simulink model "target_generation_lib_test"  (R2018b)
settings: Solver=VariableStepAuto  StartTime=0.0  StopTime=10.0  RelTol=1e-3
undefined symbols (not defined in the file): fswParams
libraries: sharedutil x2, sharedtransform x2, target_gen_lib x1
settings Model: Creator=taylorreynolds  LastModifiedBy=taylorreynolds

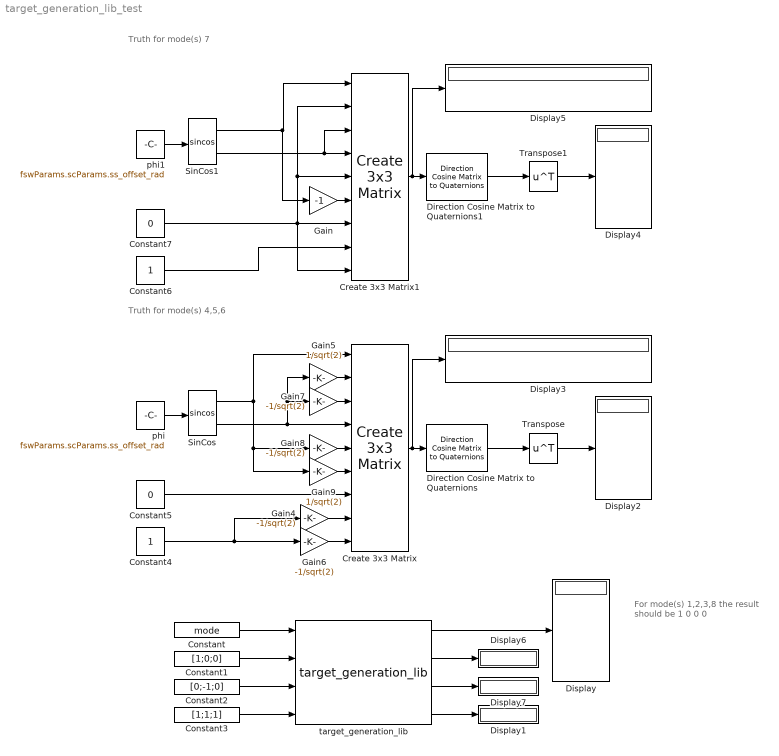
== system target_generation_lib_test ==
  note: For mode(s) 1,2,3,8
      | the result should be
      | 1
      | 0
      | 0
      | 0
  note: Truth for mode(s) 7
  note: Truth for mode(s) 4,5,6
  Constant : Constant  Value=mode  mask{mode=6}
      mask prompts: mode "Choose gnc_mode"
      mask TypeOptions mode: 1 | 2 | 3 | 4 | 5 | 6 | 7 | 8
  Constant1 : Constant  Value=[1;0;0]
  Constant2 : Constant  Value=[0;-1;0]
  Constant3 : Constant  Value=[1;1;1]
  Constant4 : Constant
  Constant5 : Constant  Value=0
  Constant6 : Constant
  Constant7 : Constant  Value=0
  Create 3x3 Matrix : sharedutil/Create 3x3 Matrix  aMode=aMode
  Create 3x3 Matrix1 : sharedutil/Create 3x3 Matrix  aMode=aMode
  Direction Cosine Matrix to Quaternions : sharedtransform/Direction Cosine Matrix  to Quaternions  aMode=0  action=None  tolerance=eps(2)
      settings: SourceProductName=Aerospace Blockset  SourceProductBaseCode=AE
  Direction Cosine Matrix to Quaternions1 : sharedtransform/Direction Cosine Matrix  to Quaternions  aMode=0  action=None  tolerance=eps(2)
      settings: SourceProductName=Aerospace Blockset  SourceProductBaseCode=AE
  Display{,1..7} (8 alike) : Display
  Gain : Gain  Gain=-1
  Gain{4,6..8} (4 alike) : Gain  Gain=-1/sqrt(2)
  Gain5 : Gain  Gain=1/sqrt(2)
  Gain9 : Gain  Gain=1/sqrt(2)
  SinCos : Trigonometry  Operator=sincos
  SinCos1 : Trigonometry  Operator=sincos
  Transpose : Math  Operator=transpose  SaturateOnIntegerOverflow=on
  Transpose1 : Math  Operator=transpose  SaturateOnIntegerOverflow=on
  phi : Constant  Value=fswParams.scParams.ss_offset_rad
  phi1 : Constant  Value=fswParams.scParams.ss_offset_rad
  target_generation_lib : target_gen_lib/target_generation_lib  SystemSampleTime=-1
  wires:
  target_generation_lib/1 -> Display/1
  target_generation_lib/4 -> Display1/1
  Constant/1 -> target_generation_lib/1
  Constant1/1 -> target_generation_lib/2
  Constant2/1 -> target_generation_lib/3
  Constant3/1 -> target_generation_lib/4
  Create 3x3 Matrix/1 -> Display3/1, Direction Cosine Matrix to Quaternions/1
  SinCos/1 -> Gain9/1, Gain8/1, Create 3x3 Matrix/1
  Constant4/1 -> Gain4/1, Gain6/1
  Transpose/1 -> Display2/1
  Direction Cosine Matrix to Quaternions/1 -> Transpose/1
  SinCos/2 -> Gain7/1, Gain5/1, Create 3x3 Matrix/4
  Gain8/1 -> Create 3x3 Matrix/5
  Gain7/1 -> Create 3x3 Matrix/3
  Gain4/1 -> Create 3x3 Matrix/8
  Constant5/1 -> Create 3x3 Matrix/7
  Gain5/1 -> Create 3x3 Matrix/2
  Gain6/1 -> Create 3x3 Matrix/9
  phi/1 -> SinCos/1
  Gain9/1 -> Create 3x3 Matrix/6
  Create 3x3 Matrix1/1 -> Display5/1, Direction Cosine Matrix to Quaternions1/1
  SinCos1/1 -> Gain/1, Create 3x3 Matrix1/1
  Constant6/1 -> Create 3x3 Matrix1/8
  Transpose1/1 -> Display4/1
  Direction Cosine Matrix to Quaternions1/1 -> Transpose1/1
  phi1/1 -> SinCos1/1
  Constant7/1 -> Create 3x3 Matrix1/9, Create 3x3 Matrix1/7, Create 3x3 Matrix1/5, Create 3x3 Matrix1/2
  SinCos1/2 -> Create 3x3 Matrix1/4, Create 3x3 Matrix1/3
  Gain/1 -> Create 3x3 Matrix1/6
  target_generation_lib/2 -> Display6/1
  target_generation_lib/3 -> Display7/1
